simulink library "xpcdiamondlib"  (Simulink 6.0)
settings: Solver=ode45  SolverMode=SingleTasking  StartTime=0.0  StopTime=10.0  RelTol=1e-3
values from neighbouring files (symbols this model uses):
  channel = Channels(i)    [madadvpcl812.m]    (also in madrtddm64x0.m = round(channel); madsbsiphiadc.m = round(channel); madueipd2mfx.m = round(channel); mdaadvpcl812.m)
undefined symbols (not defined in the file or in its folder): maddiamondmm, maddiamondmm32, maddiamondmm32frame, maddsmm16at, madprometheus, mdadiamondmm, mdadiamondmmx, mdadsmm16at, mdaprometheus, mdidiamondmm, mdiodiamondquartz, mdiodsmm, mdodiamondmm, mdsrubymm, mdsrubymm1612, mdsrubymm416, misa8255
libraries: xpcmeasurementcomputinglib x12
(part 1 of 2)
settings Model: Creator=adowd  LastModifiedBy=gweast
settings DataIOCC: SignalLoggingName=logsOut
settings OptimizationCC: BooleanDataType=off
settings DebuggingCC: CheckExecutionContextPreStartOutputMsg=on  CheckExecutionContextRuntimeOutputMsg=on  SolverPrmCheckMsg=none
settings HardwareCC: TargetUnknown=on

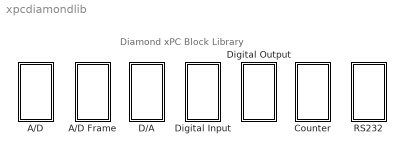
== system xpcdiamondlib ==
  note: Diamond xPC Block Library
  A/D : Subsystem  PropExecContextAcrossSSBoundary=on
  A/D Frame : Subsystem  PropExecContextAcrossSSBoundary=on
  Counter : Subsystem  PropExecContextAcrossSSBoundary=on
  D/A : Subsystem  PropExecContextAcrossSSBoundary=on
  Digital Input : Subsystem  PropExecContextAcrossSSBoundary=on
  Digital Output : Subsystem  PropExecContextAcrossSSBoundary=on
  RS232 : Subsystem  PropExecContextAcrossSSBoundary=on

== system xpcdiamondlib/A/D ==
  "MM " : S-Function  InitFcn=maddiamondmm(1)  FunctionName=addiamondmm  Parameters="numChans,  gain, offset, showStatus, sampleTime, baseDec"  mask(addiamondmm){numChans=1, range=-5V to 5V, coupling=16 single-ended channels, showStatus=off, sampleTime=0.001, base=0x300}
      mask prompts: numChans "Number of channels:"; showStatus "Show error status output (E)"; sampleTime "Sample time:"; base "Base address (e.g. 0x300):"
      mask help:
      | MM
      | Diamond
      | Analog Input
      mask init:
      | phase = 2;
      | [gain, offset, baseDec, maskDisplay, maskDescription] = maddiamondmm(phase, numChans, range, coupling, showStatus, sampleTime, base);
      | set_param(gcb, 'MaskDescription', maskDescription);
      | set_param(gcb, 'MaskDisplay', maskDisplay);
      mask Help: helpview(fullfile(docroot, 'mapfiles', 'xpc.map'), 'Diamond_MM_AD')
      mask StyleString: edit,popup(0 to 10V|0 to 5V|0 to 2V|0 to 1V|0 to Custom|-10V to 10V|-5V to 5V|-2.5V to 2.5V|-1V to 1V|-0.5V to 0.5V|-Custom to Custom),popup(16 single-ended channels|8 differential channels),checkbox,edit,edit
      mask Display: disp('MM\nDiamond\nAnalog Input'); port_label('output', 1, '1');
  "MM-16-AT " : S-Function  InitFcn=maddsmm16at(1)  FunctionName=addsmm16at  Parameters="firstChan, numChans,  gain, offset, rangeCode, showStatus, sampleTime, baseDec"  mask(addiamondmm16at){firstChan=1, numChans=1, range=-5V to 5V, coupling=16 single-ended channels, showStatus=off, sampleTime=0.001, base=0x300}
      mask prompts: firstChan "First channel:"; numChans "Number of channels:"; showStatus "Show error status output (E)"; sampleTime "Sample time:"; base "Base address (e.g. 0x300):"
      mask help:
      | MM-16-AT
      | Diamond
      | Analog Input
      mask init:
      | phase = 2;
      | [gain, offset, rangeCode, baseDec, maskDisplay, maskDescription] = maddsmm16at(phase, firstChan, numChans, range, coupling, showStatus, sampleTime, base);
      | set_param(gcb, 'MaskDescription', maskDescription);
      | set_param(gcb, 'MaskDisplay', maskDisplay);
      mask Help: helpview(fullfile(docroot, 'mapfiles', 'xpc.map'), 'Diamond_MM-16-AT_AD')
      mask StyleString: edit,edit,popup(0 to 10V|0 to 5V|0 to 2.5V|0 to 1.25V|-10V to 10V|-5V to 5V|-2.5V to 2.5V|-1.25V to 1.25V|-0.625V to 0.625V),popup(16 single-ended channels|8 differential channels),checkbox,edit,edit
      mask Display: disp('MM-16-AT\nDiamond\nAnalog Input'); port_label('output', 1, '1');
  "MM-32 " : S-Function  InitFcn=maddiamondmm32(1)  FunctionName=addiamondmm32  Parameters="firstChan, numChans,  range,  sampleTime, baseDec"  mask(addiamondmm32){configuration=1-32 SE, firstChan=1, numChans=1, range=-10V to +10V, sampleTime=0.001, base=0x300}
      mask prompts: configuration "Channel configuration"; firstChan "First channel number:"; numChans "Number of channels:"; sampleTime "Sample time:"; base "Base address (e.g. 0xd000):"
      mask help:
      | MM-32
      | Diamond
      | Analog Input
      mask init:
      | phase = 2;
      | [baseDec, maskDisplay, maskDescription] = maddiamondmm32(phase, configuration, firstChan, numChans, range, base);
      | set_param(gcb, 'MaskDescription', maskDescription);
      | set_param(gcb, 'MaskDisplay', maskDisplay);
      mask Help: helpview(fullfile(docroot, 'mapfiles', 'xpc.map'), 'Diamond_MM-32_AD')
      mask StyleString: popup(1-32 SE|1-16 DI|1-8 SE  9-16 DI  17-24 SE ),edit,edit,popup(-10V to +10V|-5V to 5V|-2.5V to +2.5V|-1.25V to +1.25V|-0.625V to +0.625V|0 to 10V|0 to 5V|0 to 2.5V|0 to 1.25V),edit,edit
      mask Display: disp('MM-32\nDiamond\nAnalog Input'); port_label('output', 1, '1');
  "Prometheus " : S-Function  InitFcn=madprometheus(1)  FunctionName=adprometheus  Parameters=firstChannel, numChannels, gain, offset, control, sampleTime, baseDec, showStatus  mask(adprometheus){firstChannel=1, numChannels=1, range=+-10V, mux=Single Ended (16 channel), showStatus=off, sampleTime=.001, base=0x280}
      mask prompts: firstChannel "First channel:"; numChannels "Number of channels:"; range "Range (J13 setting)"; mux "Input coupling (J13 setting)"; showStatus "Show error status output port (E)"; sampleTime "Sample time:"; base "Base address (e.g. 0x280):"
      mask help:
      | Prometheus
      | Diamond
      | Analog Input
      mask init:
      | phase = 2;
      | [gain, offset, control, baseDec, maskDisplay, maskDescription] = madprometheus(phase, firstChannel, numChannels, range, mux, base, showStatus);
      | set_param(gcb, 'MaskDescription', maskDescription);
      | set_param(gcb, 'MaskDisplay', maskDisplay);
      mask Help: helpview(fullfile(docroot, 'mapfiles', 'xpc.map'), 'Diamond_Prometheus_AD')
      mask StyleString: edit,edit,popup(+-10V|+-5V|+-2.5V|+-1.25V|0-10V|0-5V|0-2.5V),popup(Single Ended (16 channel)|Differential (8 channel)),checkbox,edit,edit
      mask Display: disp('Prometheus\nDiamond\nAnalog Input'); port_label('output', 1, '1');

== system xpcdiamondlib/A/D Frame ==
  "MM-32 Frame " : S-Function  InitFcn=maddiamondmm32frame(1);  StartFcn=maddiamondmm32frame(1)  FunctionName=addiamondmm32frame  Parameters="range,  firstChan, numChans,  numScans, scanInterval, freq12, count1, count2, outSigType, baseDec"  mask(addiamondmm32){configuration=1-32 Single-Ended, outSigType=Vector, range=-10V to +10V, firstChan=1, numChans=1, numScans=2, scanInterval=5 microseconds, scanTime=0.001, base=0x300}
      mask prompts: configuration "Channel configuration"; outSigType "Output signal type"; firstChan "First channel number:"; numChans "Number of channels:"; numScans "Number of scans per frame:"; scanInterval "Interval between conversions within a scan:"; scanTime "Interval between scans (seconds):"; base "Base address (e.g. 0x300):"
      mask help:
      | MM-32 Frame
      | Diamond
      | Analog Input
      mask init:
      | phase = 2;
      | [freq12, count1, count2, baseDec, maskDisplay, maskDescription] = ...
      | 	maddiamondmm32frame(phase, configuration, firstChan, numChans, numScans, scanInterval, scanTime, base);
      | set_param(gcb, 'MaskDescription', maskDescription);
      | set_param(gcb, 'MaskDisplay', maskDisplay);
      mask Help: helpview(fullfile(docroot, 'mapfiles', 'xpc.map'), 'Diamond_MM-32-Frame_AD')
      mask StyleString: popup(1-32 Single-Ended|1-16 Differential|1-8 and 17-24 Single-Ended;  9-16 Differential),popup(Vector|Frame),popup(-10V to +10V|-5V to 5V|-2.5V to +2.5V|-1.25V to +1.25V|-0.625V to +0.625V|0 to 10V|0 to 5V|0 to 2.5V|0 to 1.25V),edit,edit,edit,popup(5 microseconds|10 microseconds|15 microseconds|20 microseconds),edit,edit
      mask Display: disp('MM-32 Frame\nDiamond\nAnalog Input'); port_label('output', 1, '1');

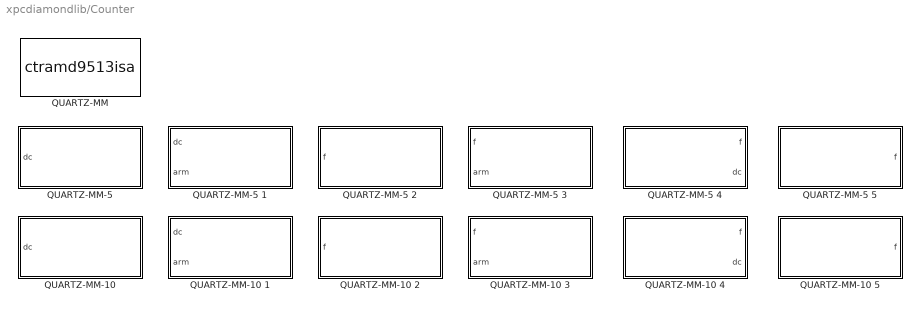
== system xpcdiamondlib/Counter ==
  "QUARTZ-MM " : S-Function  FunctionName=ctramd9513isa  Parameters=io, mm, cms, initir, ir, termir, ts, baseAddress  mask(quartzmm10){mastermode=[], countermode=[], init=[], commands=[], term=[], ts=0.001, baseAddress='0x300'}
      mask prompts: mastermode "Master mode structure:"; countermode "Counter mode structure:"; init "Initialization command structure:"; commands "Runtime command structure:"; term "Termination command structure:"; ts "Sample time:"; baseAddress "9513 chip base address (i.e. 0xd000):"
      mask help:
      | QUARTZ-MM
      | Diamond Systems
      | AMD9513 Counter
      mask init:
      | baseAddress=hex2dec(baseAddress(3:end));
      | [io,mm, cms, initir, ir, termir]=mamd9513parse(mastermode, countermode, init, commands, term);
      mask Help: helpview(fullfile(docroot, 'mapfiles', 'xpc.map'), 'Diamond_QUARTZ-MM_Counter')
      mask Display: disp('AMD9513\nCounter')
  "QUARTZ-MM-10 " : Subsystem  PropExecContextAcrossSSBoundary=on  mask(PWM){counterin=1, freq_base=F1=4MHz, freq=0.001, seq=High - Low, level=High, Ts=0.001, baseAddress=0x300}
      mask prompts: counterin "Counter:"; freq_base "Frequency base:"; freq "Relative output frequency:"; seq "Level sequence of square wave:"; level "Level when disarmed:"; Ts "Sample time:"; baseAddress "Base address (i.e. 0xd000):"
      mask help:
      | QUARTZ-MM-10
      | Diamond Systems
      | PWM
      mask init:
      | init_arm=0;
      | initduty=0.5;
      | counter=counterin;
      | if counter>5
      | counter=counter-5;
      | baseAddress=['0x',dec2hex(hex2dec(baseAddress(3:end))+4)];
      | end;
      | [MasterMode, CounterMode, Init, Runtime, Term] =pwmarm_amd9513(counter, freq_base, freq, initduty, level, init_arm);
      | level=level-1;
      | seq=seq-1;
      mask Help: helpview(fullfile(docroot, 'mapfiles', 'xpc.map'), 'Diamond_QUARTZ-MM-10_Counter')
      mask StyleString: popup(1|2|3|4|5|6|7|8|9|10),popup(F1=4MHz|F2=400KHz|F3=40kHz|F4=4kHz|F5=400Hz),edit,popup(High - Low|Low- High),popup(Low|High),edit,edit
      mask Display: text(0.95,0.75,'QUARTZ-MM-10','horizontalAlignment','right');text(0.95,0.50,'Diamond Sys','horizontalAlignment','right');text(0.95,0.25,'PWM','horizontalAlignment','right');port_label('input',1,[num2str(counterin),' (dc)'] );
  QUARTZ-MM-10 1 : Subsystem  PropExecContextAcrossSSBoundary=on  mask(PWM){counterin=1, freq_base=F1=4MHz, freq=0.001, seq=High - Low, level=High, Ts=0.001, baseAddress=0x300}
      mask prompts: counterin "Counter:"; freq_base "Frequency base:"; freq "Relative output frequency:"; seq "Level sequence of square wave:"; level "Level when disarmed:"; Ts "Sample time:"; baseAddress "Base address (i.e. 0xd000):"
      mask help:
      | QUARTZ-MM-10
      | Diamond Systems
      | PWM & ARM
      mask init: same as xpcdiamondlib/Counter/QUARTZ-MM-10 
      mask Help: helpview(fullfile(docroot, 'mapfiles', 'xpc.map'), 'Diamond_QUARTZ-MM-10-1_Counter')
      mask StyleString: popup(1|2|3|4|5|6|7|8|9|10),popup(F1=4MHz|F2=400KHz|F3=40kHz|F4=4kHz|F5=400Hz),edit,popup(High - Low|Low- High),popup(Low|High),edit,edit
      mask Display: text(0.95,0.75,'QUARTZ-MM-10','horizontalAlignment','right');text(0.95,0.50,'Diamond Sys','horizontalAlignment','right');text(0.95,0.25,'PWM & ARM','horizontalAlignment','right');port_label('input',1,[num2str(counterin),' (dc)'] );port_label('input',2,[num2str(counterin),' (arm)'] );
  QUARTZ-MM-10 2 : Subsystem  PropExecContextAcrossSSBoundary=on  mask(PWM){counterin=1, freq_base=F1=4MHz, duty=0.001, seq=High - Low, level=High, Ts=0.001, baseAddress=0x300}
      mask prompts: counterin "Counter:"; freq_base "Frequency base:"; duty "Output duty cycle:"; seq "Level sequence of square wave:"; level "Level when disarmed:"; Ts "Sample time:"; baseAddress "Base address (i.e. 0xd000):"
      mask help:
      | QUARTZ-MM-10
      | Diamond Systems
      | FM
      mask init:
      | init_arm=0;
      | initfreq=0.005;
      | counter=counterin;
      | if counter>5
      | counter=counter-5;
      | baseAddress=['0x',dec2hex(hex2dec(baseAddress(3:end))+4)];
      | end;
      | [MasterMode, CounterMode, Init, Runtime, Term] =fmarm_amd9513(counter, freq_base, duty, initfreq, level, init_arm);
      | level=level-1;
      | seq=seq-1;
      mask Help: helpview(fullfile(docroot, 'mapfiles', 'xpc.map'), 'Diamond_QUARTZ-MM-10-2_Counter')
      mask StyleString: popup(1|2|3|4|5|6|7|8|9|10),popup(F1=4MHz|F2=400KHz|F3=40kHz|F4=4kHz|F5=400Hz),edit,popup(High - Low|Low- High),popup(Low|High),edit,edit
      mask Display: text(0.95,0.75,'QUARTZ-MM-10','horizontalAlignment','right');text(0.95,0.50,'Diamond Sys','horizontalAlignment','right');text(0.95,0.25,'FM','horizontalAlignment','right');port_label('input',1,[num2str(counterin),' (f)'] );
  QUARTZ-MM-10 3 : Subsystem  PropExecContextAcrossSSBoundary=on  mask(FM){counterin=1, freq_base=F1=4MHz, duty=0.001, seq=High - Low, level=High, Ts=0.001, baseAddress=0x300}
      mask prompts: counterin "Counter:"; freq_base "Frequency base:"; duty "Output duty cycle:"; seq "Level sequence of square wave:"; level "Level when disarmed:"; Ts "Sample time:"; baseAddress "Base address (i.e. 0xd000):"
      mask help:
      | QUARTZ-MM-10
      | Diamond Systems
      | FM & ARM
      mask init: same as xpcdiamondlib/Counter/QUARTZ-MM-10 2
      mask Help: helpview(fullfile(docroot, 'mapfiles', 'xpc.map'), 'Diamond_QUARTZ-MM-10-3_Counter')
      mask StyleString: popup(1|2|3|4|5|6|7|8|9|10),popup(F1=4MHz|F2=400KHz|F3=40kHz|F4=4kHz|F5=400Hz),edit,popup(High - Low|Low- High),popup(Low|High),edit,edit
      mask Display: text(0.95,0.75,'QUARTZ-MM-10','horizontalAlignment','right');text(0.95,0.50,'Diamond Sys','horizontalAlignment','right');text(0.95,0.25,'FM & ARM','horizontalAlignment','right');port_label('input',1,[num2str(counterin),' (f)'] );port_label('input',2,[num2str(counterin),' (arm)'] );
  QUARTZ-MM-10 4 : Subsystem  PropExecContextAcrossSSBoundary=on  mask(PWMcap){counterin=1&2, freq_base=F1=4MHz, Ts=0.001, baseAddress=0x300}
      mask prompts: counterin "Counter:"; freq_base "Frequency base:"; Ts "Sample time:"; baseAddress "Base address (i.e. 0xd000):"
      mask help:
      | QUARTZ-MM-10
      | Diamond Systems
      | PWM capture
      mask init:
      | counter = counterin;
      | counterdisp = counterin;
      | if counter > 4
      | counter = counter - 4;
      | counterdisp = counterdisp + 1;
      | baseAddress=['0x',dec2hex(hex2dec(baseAddress(3:end))+4)];
      | end;
      | [MasterMode, CounterMode, Init, Runtime, Term] =pwmcap_amd9513(counter, freq_base);
      mask Help: helpview(fullfile(docroot, 'mapfiles', 'xpc.map'), 'Diamond_QUARTZ-MM-10-4_Counter')
      mask StyleString: popup(1&2|2&3|3&4|4&5|6&7|7&8|8&9|9&10),popup(F1=4MHz|F2=400KHz|F3=40kHz|F4=4kHz|F5=400Hz),edit,edit
      mask Display: text(0.05,0.75,'QUARTZ-MM-10','horizontalAlignment','left');text(0.05,0.50,'Diamond Sys','horizontalAlignment','left');text(0.05,0.25,'PWM capture','horizontalAlignment','left');port_label('output',1,[num2str(counterdisp),' (f)'] );port_label('output',2,[num2str(counterdisp+1),' (dc)'] );
  QUARTZ-MM-10 5 : Subsystem  PropExecContextAcrossSSBoundary=on  mask(FREQcap){counterin=1, freq_base=F1=4MHz, Ts=0.001, baseAddress=0x300}
      mask prompts: counterin "Counter:"; freq_base "Frequency base:"; Ts "Sample time:"; baseAddress "Base address (i.e. 0xd000):"
      mask help:
      | QUARTZ-MM-10
      | Diamond Systems
      | Frequency capture
      mask init:
      | counter=counterin;
      | if counter>5
      | counter=counter-5;
      | baseAddress=['0x',dec2hex(hex2dec(baseAddress(3:end))+4)];
      | end;
      | [MasterMode, CounterMode, Init, Runtime, Term] =freqcap_amd9513(counter, freq_base);
      mask Help: helpview(fullfile(docroot, 'mapfiles', 'xpc.map'), 'Diamond_QUARTZ-MM-10-5_Counter')
      mask StyleString: popup(1|2|3|4|5|6|7|8|9|10),popup(F1=4MHz|F2=400KHz|F3=40kHz|F4=4kHz|F5=400Hz),edit,edit
      mask Display: text(0.05,0.75,'QUARTZ-MM-10','horizontalAlignment','left');text(0.05,0.50,'Diamond Sys','horizontalAlignment','left');text(0.05,0.25,'Freq. capture','horizontalAlignment','left');port_label('output',1,[num2str(counterin),' (f)'] );
  "QUARTZ-MM-5 " : Subsystem  PropExecContextAcrossSSBoundary=on  mask(PWM){counterin=1, freq_base=F1=4MHz, freq=0.001, seq=High - Low, level=High, Ts=0.001, baseAddress=0x300}
      mask prompts: counterin "Counter:"; freq_base "Frequency base:"; freq "Relative output frequency:"; seq "Level sequence of square wave:"; level "Level when disarmed:"; Ts "Sample time:"; baseAddress "Base address (i.e. 0xd000):"
      mask help:
      | QUARTZ-MM-5
      | Diamond Systems
      | PWM
      mask init: same as xpcdiamondlib/Counter/QUARTZ-MM-10 
      mask Help: helpview(fullfile(docroot, 'mapfiles', 'xpc.map'), 'Diamond_QUARTZ-MM-5_Counter')
      mask StyleString: popup(1|2|3|4|5),popup(F1=4MHz|F2=400KHz|F3=40kHz|F4=4kHz|F5=400Hz),edit,popup(High - Low|Low- High),popup(Low|High),edit,edit
      mask Display: text(0.95,0.75,'QUARTZ-MM-5','horizontalAlignment','right');text(0.95,0.50,'Diamond Sys','horizontalAlignment','right');text(0.95,0.25,'PWM','horizontalAlignment','right');port_label('input',1,[num2str(counterin),' (dc)'] );
  QUARTZ-MM-5 1 : Subsystem  PropExecContextAcrossSSBoundary=on  mask(PWM){counterin=1, freq_base=F1=4MHz, freq=0.001, seq=High - Low, level=High, Ts=0.001, baseAddress=0x300}
      mask prompts: counterin "Counter:"; freq_base "Frequency base:"; freq "Relative output frequency:"; seq "Level sequence of square wave:"; level "Level when disarmed:"; Ts "Sample time:"; baseAddress "Base address (i.e. 0xd000):"
      mask help:
      | QUARTZ-MM-5
      | Diamond Systems
      | PWM & ARM
      mask init: same as xpcdiamondlib/Counter/QUARTZ-MM-10 
      mask Help: helpview(fullfile(docroot, 'mapfiles', 'xpc.map'), 'Diamond_QUARTZ-MM-5-1_Counter')
      mask StyleString: popup(1|2|3|4|5),popup(F1=4MHz|F2=400KHz|F3=40kHz|F4=4kHz|F5=400Hz),edit,popup(High - Low|Low- High),popup(Low|High),edit,edit
      mask Display: text(0.95,0.75,'QUARTZ-MM-5','horizontalAlignment','right');text(0.95,0.50,'Diamond Sys','horizontalAlignment','right');text(0.95,0.25,'PWM & ARM','horizontalAlignment','right');port_label('input',1,[num2str(counterin),' (dc)'] );port_label('input',2,[num2str(counterin),' (arm)'] );
  QUARTZ-MM-5 2 : Subsystem  PropExecContextAcrossSSBoundary=on  mask(PWM){counterin=1, freq_base=F1=4MHz, duty=0.001, seq=High - Low, level=High, Ts=0.001, baseAddress=0x300}
      mask prompts: counterin "Counter:"; freq_base "Frequency base:"; duty "Output duty cycle:"; seq "Level sequence of square wave:"; level "Level when disarmed:"; Ts "Sample time:"; baseAddress "Base address (i.e. 0xd000):"
      mask help:
      | QUARTZ-MM-5
      | Diamond Systems
      | FM
      mask init: same as xpcdiamondlib/Counter/QUARTZ-MM-10 2
      mask Help: helpview(fullfile(docroot, 'mapfiles', 'xpc.map'), 'Diamond_QUARTZ-MM-5-2_Counter')
      mask StyleString: popup(1|2|3|4|5),popup(F1=4MHz|F2=400KHz|F3=40kHz|F4=4kHz|F5=400Hz),edit,popup(High - Low|Low- High),popup(Low|High),edit,edit
      mask Display: text(0.95,0.75,'QUARTZ-MM-5','horizontalAlignment','right');text(0.95,0.50,'Diamond Sys','horizontalAlignment','right');text(0.95,0.25,'FM','horizontalAlignment','right');port_label('input',1,[num2str(counterin),' (f)'] );
  QUARTZ-MM-5 3 : Subsystem  PropExecContextAcrossSSBoundary=on  mask(FM){counterin=1, freq_base=F1=4MHz, duty=0.001, seq=High - Low, level=High, Ts=0.001, baseAddress=0x300}
      mask prompts: counterin "Counter:"; freq_base "Frequency base:"; duty "Output duty cycle:"; seq "Level sequence of square wave:"; level "Level when disarmed:"; Ts "Sample time:"; baseAddress "Base address (i.e. 0xd000):"
      mask help:
      | QUARTZ-MM-5
      | Diamond Systems
      | FM & ARM
      mask init: same as xpcdiamondlib/Counter/QUARTZ-MM-10 2
      mask Help: helpview(fullfile(docroot, 'mapfiles', 'xpc.map'), 'Diamond_QUARTZ-MM-5-3_Counter')
      mask StyleString: popup(1|2|3|4|5),popup(F1=4MHz|F2=400KHz|F3=40kHz|F4=4kHz|F5=400Hz),edit,popup(High - Low|Low- High),popup(Low|High),edit,edit
      mask Display: text(0.95,0.75,'QUARTZ-MM-5','horizontalAlignment','right');text(0.95,0.50,'Diamond Sys','horizontalAlignment','right');text(0.95,0.25,'FM & ARM','horizontalAlignment','right');port_label('input',1,[num2str(counterin),' (f)'] );port_label('input',2,[num2str(counterin),' (arm)'] );
  QUARTZ-MM-5 4 : Subsystem  PropExecContextAcrossSSBoundary=on  mask(PWMcap){counterin=1&2, freq_base=F1=4MHz, Ts=0.001, baseAddress=0x300}
      mask prompts: counterin "Counter:"; freq_base "Frequency base:"; Ts "Sample time:"; baseAddress "Base address (i.e. 0xd000):"
      mask help:
      | QUARTZ-MM-5
      | Diamond Systems
      | PWM capture
      mask init:
      | counter=counterin;
      | if counter>4
      | counter=counter-4;
      | baseAddress=['0x',dec2hex(hex2dec(baseAddress(3:end))+4)];
      | end;
      | [MasterMode, CounterMode, Init, Runtime, Term] =pwmcap_amd9513(counter, freq_base);
      mask Help: helpview(fullfile(docroot, 'mapfiles', 'xpc.map'), 'Diamond_QUARTZ-MM-5-4_Counter')
      mask StyleString: popup(1&2|2&3|3&4|4&5),popup(F1=4MHz|F2=400KHz|F3=40kHz|F4=4kHz|F5=400Hz),edit,edit
      mask Display: text(0.05,0.75,'QUARTZ-MM-5','horizontalAlignment','left');text(0.05,0.50,'Diamond Sys','horizontalAlignment','left');text(0.05,0.25,'PWM capture','horizontalAlignment','left');port_label('output',1,[num2str(counterin),' (f)'] );port_label('output',2,[num2str(counterin+1),' (dc)'] );
  QUARTZ-MM-5 5 : Subsystem  PropExecContextAcrossSSBoundary=on  mask(FREQcap){counterin=1, freq_base=F1=4MHz, Ts=0.001, baseAddress=0x300}
      mask prompts: counterin "Counter:"; freq_base "Frequency base:"; Ts "Sample time:"; baseAddress "Base address (i.e. 0xd000):"
      mask help:
      | QUARTZ-MM-5
      | Diamond Systems
      | Frquency capture
      mask init:
      | counter=counterin;
      | if counter>5
      | counter=counter-5;
      | baseAddress=['0x',dec2hex(hex2dec(baseAddress(3:end))+4)];
      | end;
      | [MasterMode, CounterMode, Init, Runtime, Term] =freqcap_amd9513(counter, freq_base);
      mask Help: helpview(fullfile(docroot, 'mapfiles', 'xpc.map'), 'Diamond_QUARTZ-MM-5-5_Counter')
      mask StyleString: popup(1|2|3|4|5),popup(F1=4MHz|F2=400KHz|F3=40kHz|F4=4kHz|F5=400Hz),edit,edit
      mask Display: text(0.05,0.75,'QUARTZ-MM-5','horizontalAlignment','left');text(0.05,0.50,'Diamond Sys','horizontalAlignment','left');text(0.05,0.25,'Freq. capture','horizontalAlignment','left');port_label('output',1,[num2str(counterin),' (f)'] );

== system xpcdiamondlib/D/A ==
  "MM " : S-Function  InitFcn=mdadiamondmm(1);  FunctionName=dadiamondmm  Parameters=channel, range, reset, initValue, sampleTime, baseDec  mask(dadiamondmm){channel=[1], range=[5], reset=[1], initValue=[0], sampleTime=0.001, base=0x300}
      mask prompts: channel "Channel vector:"; range "Range vector:"; reset "Reset vector:"; initValue "Initial value vector:"; sampleTime "Sample time:"; base "Base address (e.g. 0x300):"
      mask help:
      | MM
      | Diamond
      | Analog Output
      mask init:
      | phase = 2;
      | [range, reset, initValue, baseDec, maskDisplay, maskDescription] = mdadiamondmm(phase, channel, range, reset, initValue, sampleTime, base);
      | set_param(gcb, 'MaskDescription', maskDescription);
      | set_param(gcb, 'MaskDisplay', maskDisplay);
      mask Help: helpview(fullfile(docroot, 'mapfiles', 'xpc.map'), 'Diamond_MM_DA')
      mask Display: disp('MM\nDiamond\nAnalog Output'); port_label('input', 1, '1');
  "MM-16-AT " : S-Function  InitFcn=mdadsmm16at(1);  FunctionName=dadsmm16at  Parameters=channel, range, reset, initValue, sampleTime, baseDec  mask(dadiamondmm16at){channel=[1], range=0 to 5V, reset=[1], initValue=[0], sampleTime=0.001, base=0x300}
      mask prompts: channel "Channel vector:"; reset "Reset vector:"; initValue "Initial value vector:"; sampleTime "Sample time:"; base "Base address (e.g. 0x300):"
      mask help:
      | MM-16-AT
      | Diamond
      | Analog Output
      mask init:
      | phase = 2;
      | [reset, initValue, baseDec, maskDisplay, maskDescription] = mdadsmm16at(phase, channel, reset, initValue, sampleTime, base);
      | set_param(gcb, 'MaskDescription', maskDescription);
      | set_param(gcb, 'MaskDisplay', maskDisplay);
      mask Help: helpview(fullfile(docroot, 'mapfiles', 'xpc.map'), 'Diamond_MM-16-AT_DA')
      mask StyleString: edit,popup(0 to 5V|-5V to 5V),edit,edit,edit,edit
      mask Display: disp('MM-16-AT\nDiamond\nAnalog Output'); port_label('input', 1, '1');
  "MM-32 " : S-Function  InitFcn=mdadiamondmmx(1,1);  FunctionName=dadiamondmmx  Parameters=channel, range, reset, initValue, sampletime, baseaddress, boardType  mask(dadiamondmm32){channel=[1], range=+-10V, reset=[1], initValue=[0], sampletime=0.001, baseaddress=0x300}
      mask prompts: channel "Channel vector:"; range "Range vector:"; reset "Reset vector:"; initValue "Initial value vector:"; sampletime "Sample time:"; baseaddress "Base address (i.e. 0xd000):"
      mask help:
      | MM-32
      | Diamond Systems
      | Analog Output
      mask init:
      | boardType=1;
      | baseaddress1=baseaddress;
      | baseaddress=hex2dec(baseaddress(3:end));
      | [maskdisplay, maskdescription, reset, initValue]= mdadiamondmmx(2, boardType, channel, baseaddress1, reset, initValue);
      | 
      | set_param(gcb,'MaskDescription',maskdescription);
      | set_param(gcb,'MaskDisplay',maskdisplay);
      mask Help: helpview(fullfile(docroot, 'mapfiles', 'xpc.map'), 'Diamond_MM-32_DA')
      mask StyleString: edit,popup(+-10V|+-5V|0-10V|0-5V),edit,edit,edit,edit
      mask Display: disp('MM-32\nDiamond\nAnalog Output');port_label('input',1,'1');
  "Prometheus " : S-Function  InitFcn=mdaprometheus(1)  FunctionName=daprometheus  Parameters=channel, range, reset, initValue, sampleTime, baseDec, showStatus  mask(daprometheus){channel=[1], range=-10V to 10V, reset=[1], initValue=[0], showStatus=off, sampleTime=0.001, base=0x280}
      mask prompts: channel "Channel vector:"; range "Range  (J13 setting)"; reset "Reset vector:"; initValue "Initial value vector:"; showStatus "Show error status output port (E):"; sampleTime "Sample time:"; base "Base address (e.g. 0x280):"
      mask help:
      | Prometheus
      | Diamond
      | Analog Output
      mask init:
      | phase = 2;
      | [maskDisplay, maskDescription, reset, initValue, baseDec] = mdaprometheus(phase, channel, reset, initValue, sampleTime, base, showStatus);
      | set_param(gcb,'MaskDescription', maskDescription);
      | set_param(gcb,'MaskDisplay', maskDisplay);
      mask Help: helpview(fullfile(docroot, 'mapfiles', 'xpc.map'), 'Diamond_Prometheus_DA')
      mask StyleString: edit,popup(-10V to 10V|0 to 10V),edit,edit,checkbox,edit,edit
      mask Display: disp('Prometheus\nDiamond\nAnalog Output'); port_label('input', 1, '1');
  "Ruby-MM " : S-Function  InitFcn=mdsrubymm(1)  FunctionName=dadsrubymm  Parameters=channel, range0, range1, reset, initValue, st, base  mask(dsRubyMM-daout){channel=[1], range0=+-10, range1=+-10, reset=[1], initValue=[0], st=.001, baseaddress=0x300}
      mask prompts: channel "Channel vector:"; range0 "Range (channels 1-4):"; range1 "Range (channels 5-8):"; reset "Reset vector:"; initValue "Initial value vector:"; st "Sample time:"; baseaddress "Base address (i.e. 0xd000):"
      mask help:
      | Ruby-MM
      | Diamond Systems
      | Analog Output
      mask init:
      | [maskdisplay, base, reset, initValue] = mdsrubymm( 2, channel, baseaddress, reset, initValue );
      | set_param( gcb, 'MaskDisplay', maskdisplay );
      mask Help: helpview(fullfile(docroot, 'mapfiles', 'xpc.map'), 'Diamond_Ruby-MM_DA')
      mask StyleString: edit,popup(+-10|+-5|+-2.5|0-10|0-5|0-2.5),popup(+-10|+-5|+-2.5|0-10|0-5|0-2.5),edit,edit,edit,edit
      mask Display: disp('Ruby-MM\nDiamond\nAnalog Output'); port_label('input',1,'1');
  "Ruby-MM-1612 " : S-Function  InitFcn=mdsrubymm1612(1)  FunctionName=dadsrubymm1612  Parameters=channel, range, reset, initValue, sampleTime, baseDec  mask(dadsrubymm1612){channel=[1], range1=-5V to 5V, range2=-5V to 5V, reset=[1], initValue=[0], sampleTime=.001, base=0x300}
      mask prompts: channel "Channel vector:"; range1 "Range for bank 1 (channels 1-8):"; range2 "Range for bank 2 (channels 9-16):"; reset "Reset vector:"; initValue "Initial value vector:"; sampleTime "Sample time:"; base "Base address (e.g. 0x300):"
      mask help:
      | Ruby-MM-1612
      | Diamond
      | Analog Output
      mask init:
      | [maskDisplay, maskDescription, range, reset, initValue, baseDec] = mdsrubymm1612( 2, channel, range1, range2, reset, initValue, base );
      | set_param( gcb, 'MaskDisplay', maskDisplay );
      | set_param( gcb, 'maskDescription', maskDescription );
      mask Help: helpview(fullfile(docroot, 'mapfiles', 'xpc.map'), 'Diamond_Ruby-MM-1612_DA')
      mask StyleString: edit,popup(-2.5V to 2.5V|-5V to 5V|-10V to 10V|0 to 2.5V|0 to 5V|0 to 10V),popup(-2.5V to 2.5V|-5V to 5V|-10V to 10V|0 to 2.5V|0 to 5V|0 to 10V),edit,edit,edit,edit
      mask Display: disp('Ruby-MM-1612\nDiamond\nAnalog Output'); port_label('input', 1, '1');
  "Ruby-MM-416 " : S-Function  InitFcn=mdsrubymm416(1)  FunctionName=dadsrubymm416  Parameters=channel, range, reset, initValue, sampleTime, baseDec  mask(dadsrubymm416){channel=[1], range=[-5], reset=[1], initValue=[0], sampleTime=.001, base=0x300}
      mask prompts: channel "Channel vector:"; reset "Reset vector:"; initValue "Initial value vector:"; sampleTime "Sample time:"; base "Base address (e.g. 0x300):"
      mask help:
      | Ruby-MM-416
      | Diamond
      | Analog Output
      mask init:
      | [maskDisplay, maskDescription, range, reset, initValue, baseDec] = mdsrubymm416( 2, channel, range, reset, initValue, base );
      | set_param( gcb, 'MaskDisplay', maskDisplay );
      | set_param( gcb, 'maskDescription', maskDescription );
      mask Help: helpview(fullfile(docroot, 'mapfiles', 'xpc.map'), 'Diamond_Ruby-MM-416_DA')
      mask Display: disp('Ruby-MM-416\nDiamond\nAnalog Output'); port_label('input', 1, '1');

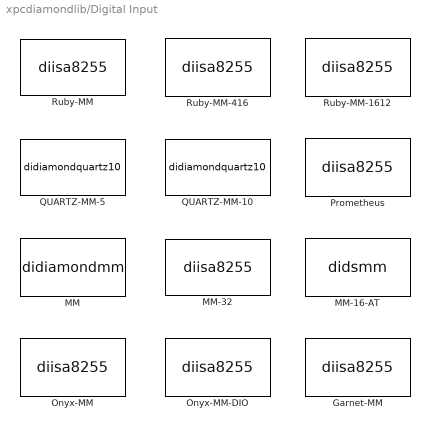
== system xpcdiamondlib/Digital Input ==
  "Garnet-MM " : S-Function  InitFcn=misa8255(1)  FunctionName=diisa8255  Parameters=channel, port, sampletime, baseaddress, control  mask(didsgarnetmm){channel=[1], port=A, chip=1, sampletime=.001, baseaddress=0x300}
      mask prompts: channel "Channel vector:"; sampletime "Sample time:"; baseaddress "Base address (e.g. 0x300):"
      mask help:
      | Garnet-MM
      | Diamond Systems
      | Digital Input
      mask init:
      | baseaddress=hex2dec(baseaddress(3:end));
      | control=155;
      | [baseaddress,control,maskdisplay,maskdescription]=misa8255(2, chip, port, channel, baseaddress);
      | set_param(gcb, 'MaskDisplay', maskdisplay);
      | set_param(gcb, 'MaskDescription', maskdescription);
      mask Help: helpview(fullfile(docroot, 'mapfiles', 'xpc.map'), 'Diamond_Garnet-MM_DIN')
      mask StyleString: edit,popup(A|B|C),popup(1|2),edit,edit
      mask Display: disp('Garnet-MM\nDiamond\nDigital Input');port_label('output',1,'1');
  "MM " : S-Function  InitFcn=mdidiamondmm(1);  FunctionName=didiamondmm  Parameters=channel, sampleTime, baseDec  mask(didiamondmm){channel=[1], sampleTime=0.001, base=0x300}
      mask prompts: channel "Channel vector:"; sampleTime "Sample time:"; base "Base address (e.g. 0x300):"
      mask help:
      | MM
      | Diamond
      | Digital Input
      mask init:
      | phase = 2;
      | [baseDec, maskDisplay, maskDescription] = mdidiamondmm(phase, channel, sampleTime, base);
      | set_param(gcb, 'MaskDisplay', maskDisplay);
      | set_param(gcb, 'MaskDescription', maskDescription);
      mask Help: helpview(fullfile(docroot, 'mapfiles', 'xpc.map'), 'Diamond_MM_DIN')
      mask Display: disp('MM\nDiamond\nDigital Input'); port_label('output', 1, '1');
  "MM-16-AT " : S-Function  InitFcn=mdiodsmm(1, 'MM-16-AT', 'input');  FunctionName=didsmm  Parameters=channel, sampleTime, baseDec  mask(didiamondmm16at){channel=[1], sampleTime=0.001, baseHex=0x300}
      mask prompts: channel "Channel vector:"; sampleTime "Sample time:"; baseHex "Base address (e.g. 0x300):"
      mask help:
      | MM-16-AT
      | Diamond
      | Digital Input
      mask init:
      | phase = 2;
      | deviceName = 'MM-16-AT';
      | direction = 'input';
      | [baseDec, maskDisplay, maskDescription] = mdiodsmm(phase, deviceName, direction, channel, sampleTime, baseHex);
      | set_param(gcb, 'MaskDisplay', maskDisplay);
      | set_param(gcb, 'MaskDescription', maskDescription);
      mask Help: helpview(fullfile(docroot, 'mapfiles', 'xpc.map'), 'Diamond_MM-16-AT_DIN')
      mask Display: disp('MM-16-AT\nDiamond\nDigital Input'); port_label('output', 1, '1');
  "MM-32 " : S-Function  InitFcn=misa8255(1)  FunctionName=diisa8255  Parameters=channel, port, sampletime, baseaddress, control  mask(didsmm32){channel=[1], port=A, chip=1, sampletime=0.001, baseaddress=0x300}
      mask prompts: channel "Channel vector:"; sampletime "Sample time:"; baseaddress "Base address (i.e. 0xd000):"
      mask help:
      | MM-32
      | Diamond Systems
      | Digital Input
      mask init:
      | baseaddress=hex2dec(baseaddress(3:end));
      | control=155;
      | boardType=16;
      | [baseaddress,control,maskdisplay,maskdescription]=misa8255(2, chip, port, channel, baseaddress);
      | set_param(gcb, 'MaskDisplay', maskdisplay);
      | set_param(gcb, 'MaskDescription', maskdescription);
      mask Help: helpview(fullfile(docroot, 'mapfiles', 'xpc.map'), 'Diamond_MM-32_DIN')
      mask StyleString: edit,popup(A|B|C),popup(1),edit,edit
      mask Display: disp('MM-32\nDiamond\nDigital Input');port_label('output',1,'1');
  "Onyx-MM " : S-Function  InitFcn=misa8255(1)  FunctionName=diisa8255  Parameters=channel, port, sampletime, baseaddress, control  mask(didsonyxmm){channel=[1], port=A, chip=1, sampletime=.001, baseaddress=0x300}
      mask prompts: channel "Channel vector:"; sampletime "Sample time:"; baseaddress "Base address (e.g. 0x300):"
      mask help:
      | Onyx-MM
      | Diamond Systems
      | Digital Input
      mask init: same as xpcdiamondlib/Digital Input/MM-32 
      mask Help: helpview(fullfile(docroot, 'mapfiles', 'xpc.map'), 'Diamond_Onyx-MM_DIN')
      mask StyleString: edit,popup(A|B|C),popup(1|2),edit,edit
      mask Display: disp('Onyx-MM\nDiamond\nDigital Input');port_label('output',1,'1');
  "Onyx-MM-DIO " : S-Function  InitFcn=misa8255(1)  FunctionName=diisa8255  Parameters=channel, port, sampletime, baseaddress, control  mask(didsonyxmmdio){channel=[1], port=A, chip=1, sampletime=.001, baseaddress=0x300}
      mask prompts: channel "Channel vector:"; sampletime "Sample time:"; baseaddress "Base address (e.g. 0x300):"
      mask help:
      | Onyx-MM-DIO
      | Diamond Systems
      | Digital Input
      mask init: same as xpcdiamondlib/Digital Input/Garnet-MM 
      mask Help: helpview(fullfile(docroot, 'mapfiles', 'xpc.map'), 'Diamond_Onyx-MM-DIO_DIN')
      mask StyleString: edit,popup(A|B|C),popup(1|2),edit,edit
      mask Display: disp('Onyx-MM-DIO\nDiamond\nDigital Input');port_label('output',1,'1');
  Prometheus : S-Function  InitFcn=misa8255(1)  FunctionName=diisa8255  Parameters=channel, port, sampletime, baseaddress, control  mask(didsprometheus){channel=[1], port=A, chip=1, sampletime=0.001, baseaddress=0x280}
      mask prompts: channel "Channel vector:"; sampletime "Sample time:"; baseaddress "Base address (e.g. 0x280):"
      mask help:
      | Prometheus
      | Diamond Systems
      | Digital Input
      mask init: same as xpcdiamondlib/Digital Input/MM-32 
      mask Help: helpview(fullfile(docroot, 'mapfiles', 'xpc.map'), 'Diamond_Prometheus_DIN')
      mask StyleString: edit,popup(A|B|C),popup(1),edit,edit
      mask Display: disp('Prometheus\nDiamond\nDigital Input');port_label('output',1,'1');
  "QUARTZ-MM-10 " : S-Function  InitFcn=mdiodiamondquartz(1);  FunctionName=didiamondquartz10  Parameters=channel, ts, baseAddress  mask(didiamondquartz10){channel=[1], ts=0.001, baseAddressIn=0x300}
      mask prompts: channel "Channel vector:"; ts "Sample time:"; baseAddressIn "Base address (i.e. 0xd000):"
      mask help:
      | Quartz-MM-10
      | Diamond
      | Digital Input
      mask init:
      | type=2;
      | baseAddress=768;
      | [baseAddress, maskdisplay,maskdescription]=mdiodiamondquartz(2, type, channel, baseAddressIn);
      | set_param(gcb,'MaskDisplay',maskdisplay);
      | set_param(gcb,'MaskDescription',maskdescription);
      mask Help: helpview(fullfile(docroot, 'mapfiles', 'xpc.map'), 'Diamond_QUARTZ-MM-10_DIN')
      mask Display: disp('Quartz-MM-10\nDiamond\nDigital Input'); port_label('output', 1, '1');
  "QUARTZ-MM-5 " : S-Function  InitFcn=mdiodiamondquartz(1);  FunctionName=didiamondquartz10  Parameters=channel, ts, baseAddress  mask(didiamondquartz5){channel=[1], ts=0.001, baseAddressIn=0x300}
      mask prompts: channel "Channel vector:"; ts "Sample time:"; baseAddressIn "Base address (i.e. 0xd000):"
      mask help:
      | Quartz-MM-5
      | Diamond
      | Digital Input
      mask init:
      | type=4;
      | baseAddress=768;
      | [baseAddress, maskdisplay,maskdescription]=mdiodiamondquartz(2, type, channel, baseAddressIn);
      | set_param(gcb,'MaskDisplay',maskdisplay);
      | set_param(gcb,'MaskDescription',maskdescription);
      mask Help: helpview(fullfile(docroot, 'mapfiles', 'xpc.map'), 'Diamond_QUARTZ-MM-5_DIN')
      mask Display: disp('Quartz-MM-5\nDiamond\nDigital Input'); port_label('output', 1, '1');
  "Ruby-MM " : S-Function  InitFcn=misa8255(1)  FunctionName=diisa8255  Parameters=channel, port, sampletime, baseaddress, control  mask(didsrubymm){channel=[1], port=A, chip=1, sampletime=0.001, baseaddress=0x300}
      mask prompts: channel "Channel vector:"; sampletime "Sample time:"; baseaddress "Base address (i.e. 0xd000):"
      mask help:
      | Ruby-MM
      | Diamond Systems
      | Digital Input
      mask init: same as xpcdiamondlib/Digital Input/Garnet-MM 
      mask Help: helpview(fullfile(docroot, 'mapfiles', 'xpc.map'), 'Diamond_Ruby-MM_DIN')
      mask StyleString: edit,popup(A|B|C),popup(1),edit,edit
      mask Display: disp('Ruby-MM\nDiamond\nDigital Input');port_label('output',1,'1');
  "Ruby-MM-1612 " : S-Function  InitFcn=misa8255(1)  FunctionName=diisa8255  Parameters=channel, port, sampletime, baseaddress, control  mask(didsrubymm1612){channel=[1], port=A, chip=1, sampletime=.001, baseaddress=0x300}
      mask prompts: channel "Channel vector:"; sampletime "Sample time:"; baseaddress "Base address (e.g. 0x300):"
      mask help:
      | Ruby-MM-1612
      | Diamond Systems
      | Digital Input
      mask init: same as xpcdiamondlib/Digital Input/MM-32 
      mask Help: helpview(fullfile(docroot, 'mapfiles', 'xpc.map'), 'Diamond_Ruby-MM-1612_DIN')
      mask StyleString: edit,popup(A|B|C),popup(1),edit,edit
      mask Display: disp('Ruby-MM-1612\nDiamond\nDigital Input');port_label('output',1,'1');
  "Ruby-MM-416 " : S-Function  InitFcn=misa8255(1)  FunctionName=diisa8255  Parameters=channel, port, sampletime, baseaddress, control  mask(didsrubymm416){channel=[1], port=A, chip=1, sampletime=.001, baseaddress=0x300}
      mask prompts: channel "Channel vector:"; sampletime "Sample time:"; baseaddress "Base address (e.g. 0x300):"
      mask help:
      | Ruby-MM-416
      | Diamond Systems
      | Digital Input
      mask init: same as xpcdiamondlib/Digital Input/MM-32 
      mask Help: helpview(fullfile(docroot, 'mapfiles', 'xpc.map'), 'Diamond_Ruby-MM-416_DIN')
      mask StyleString: edit,popup(A|B|C),popup(1),edit,edit
      mask Display: disp('Ruby-MM-416\nDiamond\nDigital Input');port_label('output',1,'1');
